simulink model "PWMdutyFreqDetection"  (R2021a)
settings: Solver=FixedStepDiscrete  StartTime=0.0  StopTime=0.2e-3  RelTol=1e-3
undefined symbols (not defined in the file): t_clk, t_clk_sig
libraries: simulink x6, hdlsllib x2
settings Model: DataTypeOverride=Off  Creator=Michael Hoerner  LastModifiedBy=micha
settings SolverCC: AlgebraicLoopSolver=TrustRegion
settings DataIOCC: LimitDataPoints=on  SaveOutput=off  SaveTime=off  ReturnWorkspaceOutputs=off
settings OptimizationCC: BlockReduction=off  ConditionallyExecuteInputs=off  DefaultParameterBehavior=Inlined  LifeSpan=inf
settings DebuggingCC: AlgebraicLoopMsg=error  SingleTaskRateTransMsg=warning  AllowSymbolicDim=off  StrictBusMsg=ErrorOnBusTreatedAsVector  SFUnexpectedBacktrackingDiag=warning  SFNoUnconditionalDefaultTransitionDiag=warning  SFExecutionAtInitializationDiag=none  SFMachineParentedDataDiag=warning  ArithmeticOperatorsInVariantConditions=warning
settings HardwareCC: ProdBitPerPointer=32  ProdBitPerSizeT=32  ProdBitPerPtrDiffT=32  ProdLargestAtomicFloat=None  ProdIntDivRoundTo=Undefined  ProdEndianess=Unspecified  ProdWordSize=32  ProdHWDeviceType=ASIC/FPGA->ASIC/FPGA  ProdEqTarget=off
settings SFSimCC: SimUseLocalCustomCode=off  CustomCodeUndefinedFunction=UseInterfaceOnly
settings RTWCC: RTWUseLocalCustomCode=off
settings CodeAppCC: StateflowObjectComments=on
settings GRTTargetCC: TargetLangStandard=C89/C90 (ANSI)
settings ConfigComp: CovScope=ReferencedModels  CovMetricSettings=dw  CovSaveCumulativeToWorkspaceVar=on  CovSaveSingleToWorkspaceVar=on  CovExternalEMLEnable=off  CovSFcnEnable=off

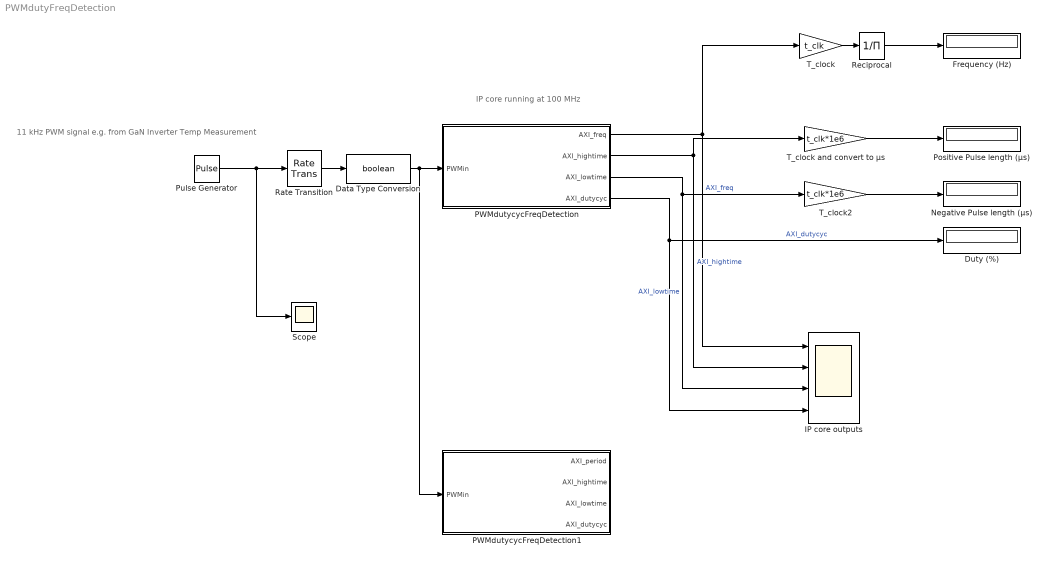
== system PWMdutyFreqDetection ==
  note: IP core running at 100 MHz
  note: 11 kHz PWM signal e.g. from GaN Inverter Temp Measurement
  Data Type Conversion : DataTypeConversion  OutDataTypeStr=boolean
  Duty (%) : Display
  Frequency (Hz) : Display
  IP core outputs : Scope  NumInputPorts=4
  Negative Pulse length (µs) : Display
  PWMdutycycFreqDetection : Subsystem  TreatAsAtomicUnit=on
  PWMdutycycFreqDetection1 : Subsystem  TreatAsAtomicUnit=on
  Positive Pulse length (µs) : Display
  Pulse Generator : DiscretePulseGenerator  PulseType=Time based  Period=t_clk_sig  PulseWidth=7.52
  Rate Transition : RateTransition  Deterministic=off  OutPortSampleTime=t_clk
  Reciprocal : Product  Inputs=/
  Scope : Scope
  T_clock : Gain  Gain=t_clk
  T_clock and convert to µs : Gain  Gain=t_clk*1e6
  T_clock2 : Gain  Gain=t_clk*1e6
  wires:
  Rate Transition/1 -> Data Type Conversion/1
  Pulse Generator/1 -> Scope/1, Rate Transition/1
  PWMdutycycFreqDetection/1(AXI_freq) -> T_clock/1, IP core outputs/1  "AXI_freq"
  PWMdutycycFreqDetection/2(AXI_hightime) -> T_clock and convert to µs/1, IP core outputs/2  "AXI_hightime"
  PWMdutycycFreqDetection/3(AXI_lowtime) -> IP core outputs/3, T_clock2/1  "AXI_lowtime"
  PWMdutycycFreqDetection/4(AXI_dutycyc) -> IP core outputs/4, Duty (%)/1  "AXI_dutycyc"
  Data Type Conversion/1 -> PWMdutycycFreqDetection1/1(PWMin), PWMdutycycFreqDetection/1(PWMin)
  T_clock/1 -> Reciprocal/1
  Reciprocal/1 -> Frequency (Hz)/1
  T_clock and convert to µs/1 -> Positive Pulse length (µs)/1
  T_clock2/1 -> Negative Pulse length (µs)/1

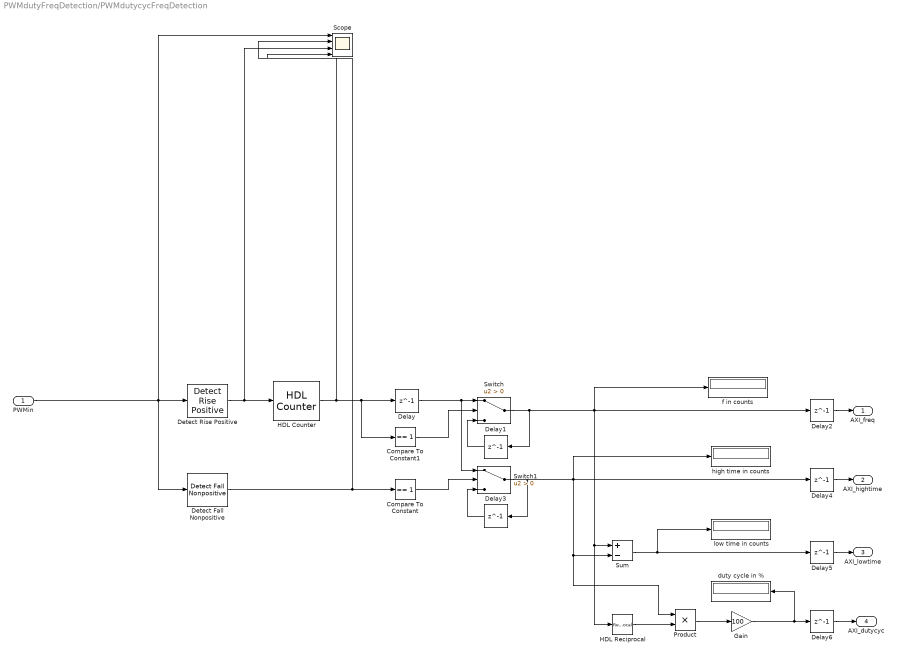
== system PWMdutyFreqDetection/PWMdutycycFreqDetection ==
  PWMin : Inport  OutDataTypeStr=boolean
  Compare To Constant : simulink/Logic and Bit Operations/Compare To Constant  relop===  const=1  OutDataTypeStr=boolean
  Compare To Constant1 : simulink/Logic and Bit Operations/Compare To Constant  relop===  const=1  OutDataTypeStr=boolean
  Delay{,1..6} (7 alike) : Delay  DelayLength=1
  Detect Fall Nonpositive : simulink/Logic and Bit Operations/Detect Fall Nonpositive  vinit=0  OutDataTypeStr=boolean
      settings: SourceProductBaseCode=SL
  Detect Rise Positive : simulink/Logic and Bit Operations/Detect Rise Positive  vinit=0  OutDataTypeStr=boolean
  Gain : Gain  Gain=100  OutDataTypeStr=fixdt(1,32,24)
  HDL Counter : hdlsllib/Sources/HDL Counter  CountType=Count limited  CountInit=1  CountStep=1  CountMax=2500000  CountFromType=Specify  CountFrom=1  CountResetPort=on  CountLoadPort=off  CountEnbPort=off  CountDirPort=off  CountHitOutputPort=off  CountDataType=Unsigned  CountWordLen=32  CountFracLen=0  CountSampTime=1
  HDL Reciprocal : Reciprocal
  Product : Product  OutDataTypeStr=fixdt(1,32,30)
  Scope : Scope  NumInputPorts=4
  Sum : Sum  Inputs=+-  AccumDataTypeStr=uint32
  Switch : Switch  Criteria=u2 > Threshold
  Switch1 : Switch  Criteria=u2 > Threshold
  duty cycle in % : Display
  f in counts : Display
  high time in counts : Display
  low time in counts : Display
  AXI_freq : Outport  VectorParamsAs1DForOutWhenUnconnected=off
  AXI_hightime : Outport  Port=2  VectorParamsAs1DForOutWhenUnconnected=off
  AXI_lowtime : Outport  Port=3  VectorParamsAs1DForOutWhenUnconnected=off
  AXI_dutycyc : Outport  Port=4  VectorParamsAs1DForOutWhenUnconnected=off
  wires:
  PWMin/1 -> Detect Fall Nonpositive/1, Scope/1, Detect Rise Positive/1
  Delay/1 -> Switch1/1, Switch/1
  Compare To Constant1/1 -> Switch/2
  Delay1/1 -> Switch/3
  Switch/1 -> Delay2/1, HDL Reciprocal/1, Sum/1, f in counts/1, Delay1/1
  Delay3/1 -> Switch1/3
  Compare To Constant/1 -> Switch1/2
  Detect Fall Nonpositive/1 -> Scope/4, Compare To Constant/1
  HDL Counter/1 -> Scope/2, Compare To Constant1/1, Delay/1
  Sum/1 -> low time in counts/1, Delay5/1
  Product/1 -> Gain/1
  HDL Reciprocal/1 -> Product/2
  Gain/1 -> Delay6/1, duty cycle in %/1
  Detect Rise Positive/1 -> Scope/3, HDL Counter/1
  Switch1/1 -> Delay4/1, Product/1, Sum/2, high time in counts/1, Delay3/1
  Delay2/1 -> AXI_freq/1
  Delay4/1 -> AXI_hightime/1
  Delay5/1 -> AXI_lowtime/1
  Delay6/1 -> AXI_dutycyc/1

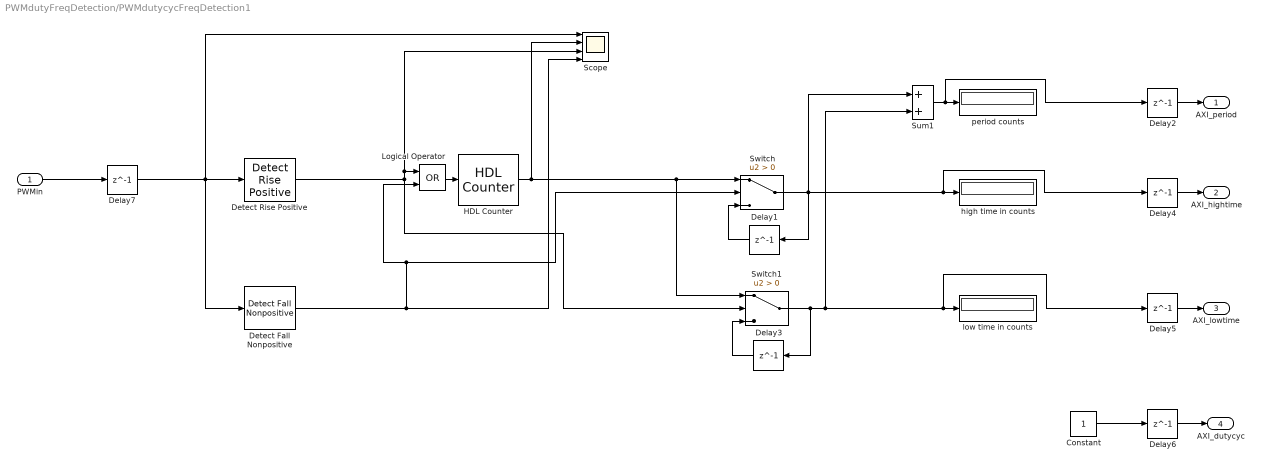
== system PWMdutyFreqDetection/PWMdutycycFreqDetection1 ==
  PWMin : Inport  OutDataTypeStr=boolean
  Constant : Constant  OutDataTypeStr=uint32  SampleTime=t_clk
  Delay{1..7} (7 alike) : Delay  DelayLength=1
  Detect Fall Nonpositive : simulink/Logic and Bit Operations/Detect Fall Nonpositive  vinit=0  OutDataTypeStr=boolean
      settings: SourceProductBaseCode=SL
  Detect Rise Positive : simulink/Logic and Bit Operations/Detect Rise Positive  vinit=0  OutDataTypeStr=boolean
  HDL Counter : hdlsllib/Sources/HDL Counter  CountType=Count limited  CountInit=1  CountStep=1  CountMax=2500000  CountFromType=Specify  CountFrom=1  CountResetPort=on  CountLoadPort=off  CountEnbPort=off  CountDirPort=off  CountHitOutputPort=off  CountDataType=Unsigned  CountWordLen=32  CountFracLen=0  CountSampTime=1
  Logical Operator : Logic  Operator=OR  AllPortsSameDT=off  OutDataTypeStr=boolean
  Scope : Scope  NumInputPorts=4
  Sum1 : Sum  AccumDataTypeStr=uint32
  Switch : Switch  Criteria=u2 > Threshold
  Switch1 : Switch  Criteria=u2 > Threshold
  high time in counts : Display
  low time in counts : Display
  period counts : Display
  AXI_period : Outport  VectorParamsAs1DForOutWhenUnconnected=off
  AXI_hightime : Outport  Port=2  VectorParamsAs1DForOutWhenUnconnected=off
  AXI_lowtime : Outport  Port=3  VectorParamsAs1DForOutWhenUnconnected=off
  AXI_dutycyc : Outport  Port=4  VectorParamsAs1DForOutWhenUnconnected=off
  wires:
  Delay7/1 -> Detect Fall Nonpositive/1, Scope/1, Detect Rise Positive/1
  Delay1/1 -> Switch/3
  Switch/1 -> Sum1/1, Delay4/1, high time in counts/1, Delay1/1
  Delay3/1 -> Switch1/3
  Switch1/1 -> Sum1/2, Delay5/1, low time in counts/1, Delay3/1
  Delay2/1 -> AXI_period/1
  Delay4/1 -> AXI_hightime/1
  Delay5/1 -> AXI_lowtime/1
  Delay6/1 -> AXI_dutycyc/1
  PWMin/1 -> Delay7/1
  Detect Rise Positive/1 -> Switch1/2, Logical Operator/1, Scope/3
  Detect Fall Nonpositive/1 -> Logical Operator/2, Switch/2, Scope/4
  HDL Counter/1 -> Switch1/1, Switch/1, Scope/2
  Logical Operator/1 -> HDL Counter/1
  Sum1/1 -> Delay2/1, period counts/1
  Constant/1 -> Delay6/1
